simulink library "lib_hierarchy"  (R2018a)
settings: Solver=ode45  StartTime=0.0  StopTime=10.0  RelTol=1e-3
settings Model: Creator=nicholas  LastModifiedBy=bneiswan
settings DataIOCC: LimitDataPoints=on  SaveFormat=Array  SignalLoggingSaveFormat=ModelDataLogs
settings OptimizationCC: BlockReduction=off  BooleanDataType=off  ExpressionDepthLimit=2147483647  LifeSpan=inf
settings DebuggingCC: SaveWithParameterizedLinksMsg=none  UnderspecifiedInitializationDetection=Classic  MergeDetectMultiDrivingBlocksExec=none  SignalResolutionControl=TryResolveAllWithWarning  FcnCallInpInsideContextMsg=warning  AllowSymbolicDim=off  StateNameClashWarn=warning  SFUnexpectedBacktrackingDiag=warning  SFNoUnconditionalDefaultTransitionDiag=warning  SFExecutionAtInitializationDiag=none
settings HardwareCC: ProdBitPerPointer=32  ProdBitPerSizeT=32  ProdBitPerPtrDiffT=32  ProdLargestAtomicFloat=None  ProdIntDivRoundTo=Undefined  ProdEndianess=Unspecified  ProdWordSize=32  ProdHWDeviceType=32-bit Generic  TargetUnknown=on
settings ModelReferenceCC: PropagateSignalLabelsOutOfModel=off
settings CodeAppCC: StateflowObjectComments=on
settings GRTTargetCC: TargetLangStandard=C89/C90 (ANSI)  GeneratePreprocessorConditionals=Disable all  CombineOutputUpdateFcns=off  GRTInterface=on
settings ConfigComp: CovMetricSettings=dw  CovHtmlReporting=on  CovSaveCumulativeToWorkspaceVar=on  CovSaveSingleToWorkspaceVar=on  CovExternalEMLEnable=off  CovSFcnEnable=off

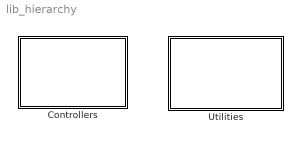
== system lib_hierarchy ==
  Controllers : Subsystem
  Utilities : Subsystem

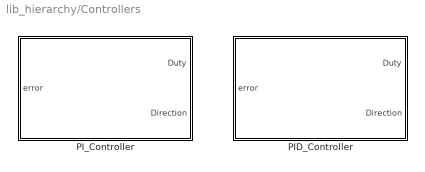
== system lib_hierarchy/Controllers ==
  PID_Controller : Subsystem  mask(PID Controller){Kp=0.3, Ki=2, Kd=0.01, Ts=0.01}
      mask prompts: Kp "Proportional Gain (Kp)"; Ki "Integral Gain (Ki)"; Kd "Derivative Gain (Kd)"; Ts "Sample Time (Ts)"
      mask help:
      | This system implements the dynamics of a discrete PID controller with a rate limiter on the integrator.
      | You must specify the proportional gain (Kp), integral gain (Ki), derivative gain (Kd), and sample time (Ts) for the system.
      mask init:
      | str1 = ['Kp = ',num2str(Kp)];
      | str2 = ['Ki = ',num2str(Ki)];
      | str3 = ['Ki = ',num2str(Kd)];
      | str4 = ['Ts = ',num2str(Ts)];
      | label = char(str1,str2,str3,str4);
      mask Display: disp(label)
  PI_Controller : Subsystem  mask(PI Controller){Kp=0.3, Ki=2, Ts=0.01}
      mask prompts: Kp "Proportional Gain (Kp)"; Ki "Integral Gain (Ki)"; Ts "Sample Time (Ts)"
      mask help:
      | This system implements the dynamics of a discrete PI controller with a rate limiter on the integrator.
      | You must specify the proportional gain (Kp), integral gain (Ki), and sample time (Ts) for the system.
      mask init:
      | str1 = ['Kp = ',num2str(Kp)];
      | str2 = ['Ki = ',num2str(Ki)];
      | str3 = ['Ts = ',num2str(Ts)];
      | label = strvcat(str1,str2,str3);
      mask Help:
      | This system implements the dynamics of a discrete PI controller with a rate limiter on the integrator.
      | The equations for the system are:  <br /><br />
      | 
      | <b>Y(k) = Yp(k) + Yi(k)</b><br />
      | Yp(k) = Kp*e(k)<br />
      | Yi(k) = Yi(k-1) + Ki*Ts*e(k)<br />
      | -1 < Yi(k) < 1<br /><br />
      | 
      | Define values for Kp, Ki, and Ts for this system.
      mask Display: disp(label)

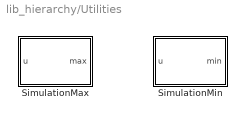
== system lib_hierarchy/Utilities ==
  SimulationMax : Subsystem  mask(Simulation Max){}
      mask help: Outputs the maximum value that the input has obtained during the simulation.
  SimulationMin : Subsystem  mask(Simulation Min){}
      mask help: Outputs the minimum value that the input has obtained during the simulation.

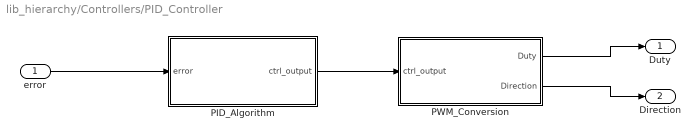
== system lib_hierarchy/Controllers/PID_Controller ==
  error : Inport  SampleTime=Ts
  PID_Algorithm : Subsystem
  PWM_Conversion : Subsystem
  Duty : Outport
  Direction : Outport  Port=2
  wires:
  error/1 -> PID_Algorithm/1(error)
  PWM_Conversion/1("Duty ") -> Duty/1
  PWM_Conversion/2(Direction) -> Direction/1
  PID_Algorithm/1(ctrl_output) -> PWM_Conversion/1(ctrl_output)

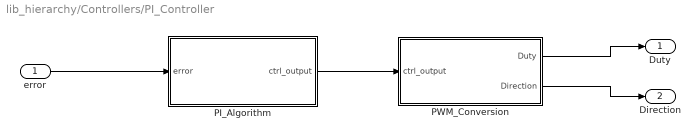
== system lib_hierarchy/Controllers/PI_Controller ==
  error : Inport  SampleTime=Ts
  PI_Algorithm : Subsystem
  PWM_Conversion : Subsystem
  Duty : Outport
  Direction : Outport  Port=2
  wires:
  PI_Algorithm/1(ctrl_output) -> PWM_Conversion/1(ctrl_output)
  PWM_Conversion/2(Direction) -> Direction/1
  PWM_Conversion/1("Duty ") -> Duty/1
  error/1 -> PI_Algorithm/1(error)

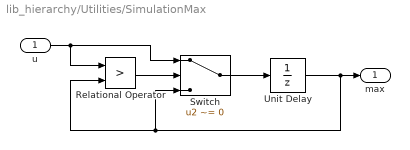
== system lib_hierarchy/Utilities/SimulationMax ==
  u : Inport
  Relational Operator : RelationalOperator  Operator=>  OutDataTypeStr=boolean  RndMeth=Nearest
  Switch : Switch  Criteria=u2 ~= 0
  Unit Delay : UnitDelay  SampleTime=-1
  max : Outport
  wires:
  Relational Operator/1 -> Switch/2
  Switch/1 -> Unit Delay/1
  u/1 -> Switch/1, Relational Operator/1
  Unit Delay/1 -> Relational Operator/2, Switch/3, max/1

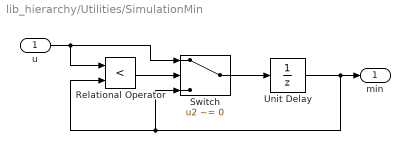
== system lib_hierarchy/Utilities/SimulationMin ==
  u : Inport
  Relational Operator : RelationalOperator  Operator=<  OutDataTypeStr=boolean  RndMeth=Nearest
  Switch : Switch  Criteria=u2 ~= 0
  Unit Delay : UnitDelay  SampleTime=-1
  min : Outport
  wires:
  Unit Delay/1 -> min/1, Switch/3, Relational Operator/2
  u/1 -> Relational Operator/1, Switch/1
  Switch/1 -> Unit Delay/1
  Relational Operator/1 -> Switch/2

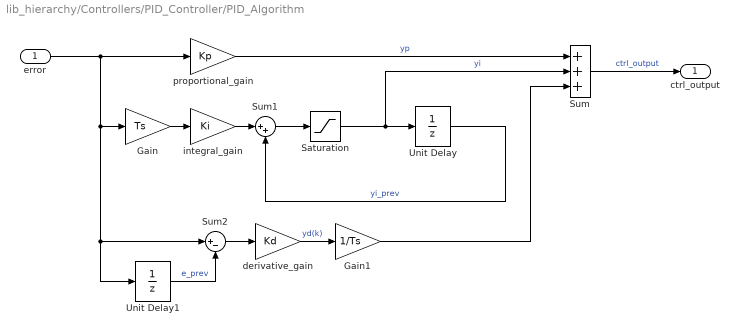
== system lib_hierarchy/Controllers/PID_Controller/PID_Algorithm ==
  error : Inport  SampleTime=Ts
      settings: AttributesFormatString=Sample time = %<SampleTime>
  Gain : Gain  Gain=Ts  SaturateOnIntegerOverflow=on  OutDataTypeStr=Inherit: Same as input  ParamDataTypeStr=Inherit: Same as input
  Gain1 : Gain  Gain=1/Ts  SaturateOnIntegerOverflow=on  OutDataTypeStr=Inherit: Same as input  ParamDataTypeStr=Inherit: Same as input
  Saturation : Saturate  UpperLimit=1  LowerLimit=-1
      settings: AttributesFormatString=Max: %<UpperLimit>\nMin: %<LowerLimit>
  Sum : Sum  Inputs=+++  SaturateOnIntegerOverflow=on  InputSameDT=on  OutDataTypeStr=Inherit: Same as first input
  Sum1 : Sum  Inputs=|++  SaturateOnIntegerOverflow=on  InputSameDT=on  OutDataTypeStr=Inherit: Same as first input
  Sum2 : Sum  Inputs=|+-  SaturateOnIntegerOverflow=on
  Unit Delay : UnitDelay  SampleTime=Ts
      settings: AttributesFormatString=yi0 = %<X0>\nSample time = %<SampleTime>
  Unit Delay1 : UnitDelay  SampleTime=Ts
      settings: AttributesFormatString=Sample Time = %<SampleTime>\nIC = %<X0>
  derivative_gain : Gain  Gain=Kd  SaturateOnIntegerOverflow=on  OutDataTypeStr=Inherit: Same as input  ParamDataTypeStr=Inherit: Same as input
  integral_gain : Gain  Gain=Ki  SaturateOnIntegerOverflow=on  OutDataTypeStr=Inherit: Same as input  ParamDataTypeStr=Inherit: Same as input
  proportional_gain : Gain  Gain=Kp  SaturateOnIntegerOverflow=on  OutDataTypeStr=Inherit: Same as input  ParamDataTypeStr=Inherit: Same as input
  ctrl_output : Outport
  wires:
  proportional_gain/1 -> Sum/1  "yp"
  integral_gain/1 -> Sum1/1
  Gain/1 -> integral_gain/1
  Unit Delay/1 -> Sum1/2  "yi_prev"
  Sum1/1 -> Saturation/1
  Saturation/1 -> Unit Delay/1, Sum/2  "yi"
  error/1 -> proportional_gain/1, Gain/1, Unit Delay1/1, Sum2/1
  Sum/1 -> ctrl_output/1  "ctrl_output"
  derivative_gain/1 -> Gain1/1  "yd(k)"
  Sum2/1 -> derivative_gain/1
  Unit Delay1/1 -> Sum2/2  "e_prev"
  Gain1/1 -> Sum/3

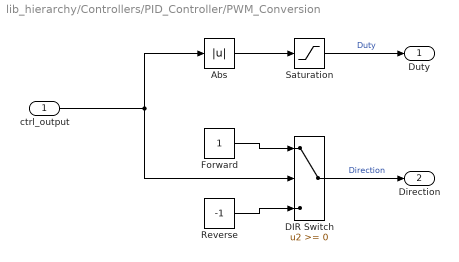
== system lib_hierarchy/Controllers/PID_Controller/PWM_Conversion ==
  ctrl_output : Inport
  Abs : Abs
  DIR Switch : Switch
      settings: AttributesFormatString=Criteria: %<Criteria>\nThreshold: %<Threshold>
  Forward : Constant  OutDataTypeStr=double
  Reverse : Constant  Value=-1  OutDataTypeStr=double
  Saturation : Saturate  UpperLimit=1  LowerLimit=0
      settings: AttributesFormatString=%<LowerLimit> < duty < %<UpperLimit>
  "Duty " : Outport
  Direction : Outport  Port=2
  wires:
  Abs/1 -> Saturation/1
  Saturation/1 -> "Duty "/1  "Duty"
  DIR Switch/1 -> Direction/1  "Direction"
  Reverse/1 -> DIR Switch/3
  Forward/1 -> DIR Switch/1
  ctrl_output/1 -> DIR Switch/2, Abs/1

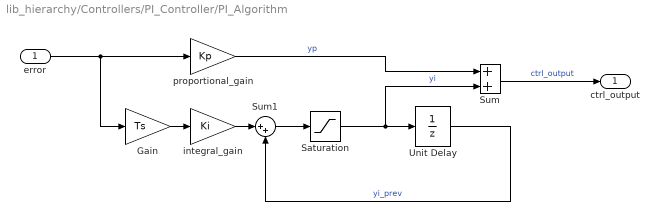
== system lib_hierarchy/Controllers/PI_Controller/PI_Algorithm ==
  error : Inport  SampleTime=Ts
      settings: AttributesFormatString=Sample time = %<SampleTime>
  Gain : Gain  Gain=Ts  SaturateOnIntegerOverflow=on  OutDataTypeStr=Inherit: Same as input  ParamDataTypeStr=Inherit: Same as input
  Saturation : Saturate  UpperLimit=1  LowerLimit=-1
      settings: AttributesFormatString=Max: %<UpperLimit>\nMin: %<LowerLimit>
  Sum : Sum  SaturateOnIntegerOverflow=on  InputSameDT=on  OutDataTypeStr=Inherit: Same as first input
  Sum1 : Sum  Inputs=|++  SaturateOnIntegerOverflow=on  InputSameDT=on  OutDataTypeStr=Inherit: Same as first input
  Unit Delay : UnitDelay  SampleTime=Ts
      settings: AttributesFormatString=yi0 = %<X0>\nSample time = %<SampleTime>
  integral_gain : Gain  Gain=Ki  SaturateOnIntegerOverflow=on  OutDataTypeStr=Inherit: Same as input  ParamDataTypeStr=Inherit: Same as input
  proportional_gain : Gain  Gain=Kp  SaturateOnIntegerOverflow=on  OutDataTypeStr=Inherit: Same as input  ParamDataTypeStr=Inherit: Same as input
  ctrl_output : Outport
  wires:
  Sum/1 -> ctrl_output/1  "ctrl_output"
  error/1 -> Gain/1, proportional_gain/1
  Saturation/1 -> Sum/2, Unit Delay/1  "yi"
  Sum1/1 -> Saturation/1
  Unit Delay/1 -> Sum1/2  "yi_prev"
  Gain/1 -> integral_gain/1
  integral_gain/1 -> Sum1/1
  proportional_gain/1 -> Sum/1  "yp"

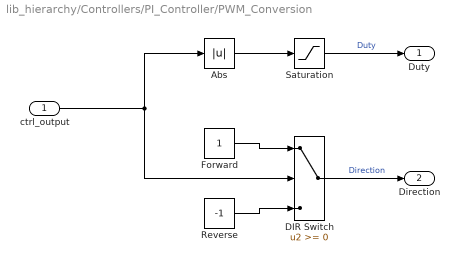
== system lib_hierarchy/Controllers/PI_Controller/PWM_Conversion ==
  ctrl_output : Inport
  Abs : Abs
  DIR Switch : Switch
      settings: AttributesFormatString=Criteria: %<Criteria>\nThreshold: %<Threshold>
  Forward : Constant  OutDataTypeStr=double
  Reverse : Constant  Value=-1  OutDataTypeStr=double
  Saturation : Saturate  UpperLimit=1  LowerLimit=0
      settings: AttributesFormatString=%<LowerLimit> < duty < %<UpperLimit>
  "Duty " : Outport
  Direction : Outport  Port=2
  wires:
  ctrl_output/1 -> Abs/1, DIR Switch/2
  Forward/1 -> DIR Switch/1
  Reverse/1 -> DIR Switch/3
  DIR Switch/1 -> Direction/1  "Direction"
  Saturation/1 -> "Duty "/1  "Duty"
  Abs/1 -> Saturation/1
